simulink model "DFPD_DA_MdlIdent"  (R2017a)
settings: Solver=VariableStepAuto  StartTime=0.0  StopTime=190  FixedStep=0.001  RelTol=1e-3  EnableMultiTasking=on
PostLoadFcn:
  | , if any(exist('dsrtsu_mdlpostloadfcn', 'file') == [2, 3, 6]), try dsrtsu_mdlpostloadfcn('Execute', bdroot); catch fprintf('Error in PostLoadFcn (dsrtsu_mdlpostloadfcn) for model "%s":\n %s\n', bdroot, lasterr); end, end,
undefined symbols (not defined in the file or in its folder): DFPD_DoubleActing, mdlPara, PASL_Models
libraries: PASL_Mechanics x3, PASL_Pneumatics x3, PASL_Components x2, PASL_Tools x2
settings Model: DSRTSU_INTERNAL_RTI_VER=500  DSRTSU_INTERNAL_RTI_TYPE=rti1401  DSRTSU_INTERNAL_RTIFPGA=90  Creator=fbwk  LastModifiedBy=fbwk
settings DataIOCC: LimitDataPoints=on  SaveFormat=Array
settings OptimizationCC: BlockReduction=off  OptimizeBlockIOStorage=off  BufferReuse=off  GlobalBufferReuse=off  ExpressionFolding=off  LocalBlockOutputs=off  LifeSpan=inf
settings DebuggingCC: SolverPrmCheckMsg=warning  SFUnexpectedBacktrackingDiag=warning  SFNoUnconditionalDefaultTransitionDiag=warning  SFExecutionAtInitializationDiag=none
settings HardwareCC: ProdBitPerPointer=32  ProdBitPerSizeT=32  ProdBitPerPtrDiffT=32  ProdLargestAtomicInteger=Integer  ProdEndianess=BigEndian  ProdWordSize=32  ProdHWDeviceType=Custom Processor->Custom  TargetIntDivRoundTo=Zero  TargetEndianess=BigEndian  TargetHWDeviceType=Custom Processor->Custom
settings ModelReferenceCC: PropagateSignalLabelsOutOfModel=off
settings SFSimCC: MATLABDynamicMemAlloc=off
settings RTWCC: SystemTargetFile=rti1005.tlc  MakeCommand=make_rti  TemplateMakefile=rti1005.tmf  Description=dSPACE DS1005 Hardware Platform
settings STFCustomTargetCC: ParMdlRefBuildCompliant=on  MatFileLogging=on  GRTInterface=off  SystemTargetFile=rti1005.tlc
settings GRTTargetCC: TargetLangStandard=C89/C90 (ANSI)  CompOptLevelCompliant=off  ConcurrentExecutionCompliant=off  CombineOutputUpdateFcns=off  CPPClassGenCompliant=off  UseToolchainInfoCompliant=off  ExtModeMexFile=noextcomm
settings ConfigComp: CovMetricSettings=dw  CovHtmlReporting=on  CovSaveCumulativeToWorkspaceVar=on  CovSaveSingleToWorkspaceVar=on  CovExternalEMLEnable=off  CovSFcnEnable=off

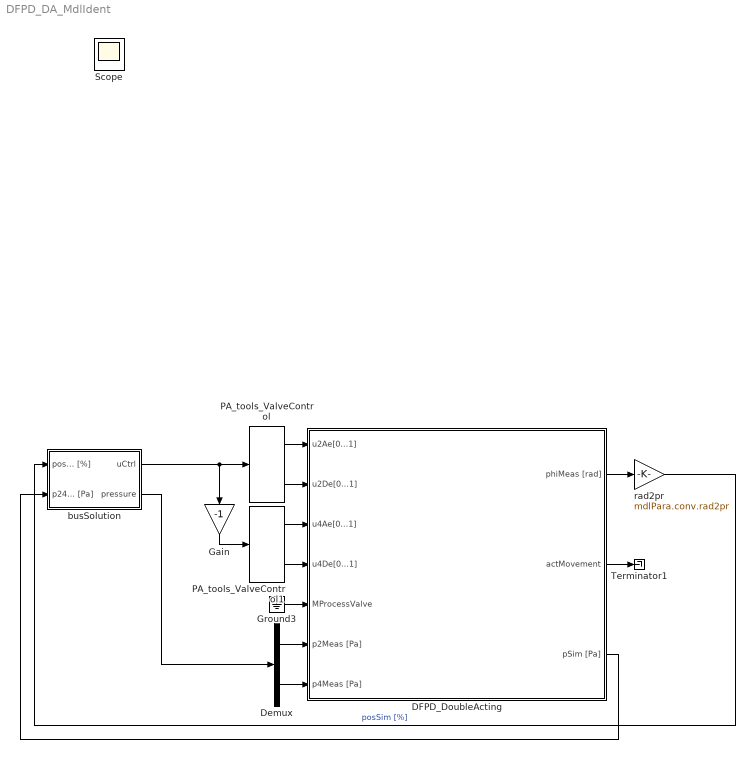
== system DFPD_DA_MdlIdent ==
  DFPD_DoubleActing : Subsystem  AncestorBlock=PASL_Models/DFPD_DoubleActing  TreatAsAtomicUnit=on  mask(Doppeltwirkender DFPD){mdlPara=mdlPara}
      mask prompts: mdlPara "Name of the parameters struct:"
      mask help:
      | Dieses Subsystem beinhaltet das Modell eines
      | doppeltwirkenden DFPDs.
      | Zur Initialisierung des Systems kann entweder
      | a) ein vorhandener Parametersatz geladen werden
      | oder
      | b) ein default Datensatz generiert werden.
      | Dabei werden die Daten des DFPD abgefragt
      | und alle aus der Konstruktion bekannten
      | Parameter entsprechend berechnet.
      |
      | !!Bisher ist das Reibungsmodell von Zahnstange
      | und Ritzel mit den Defaultwerten parametriert!!!
      |
      | 2016-09-20, lusc
      mask DialogControl Container4 Prompt: Parameter
      mask DialogControl Control5 Prompt: Parametersatz laden
      mask DialogControl Control5 Callback:
      | %% Modellparameter laden %%%%%%%%%%%%%%%%%%%%%%%%%%%%%%%%%%%%%%%%%%%%%%%%%%
      | 
      | % get mask parameters
      | maskval = get_param(gcb,'MaskValues');
      | structName = maskval{1};
      | 
      | % load parameters
      | assignin('base',structName,...
      | 	mdlPara = aux_loadMdlPara('DFPD')...
      | 	);
      | 
      | % clear section
      | clear maskval structName
      mask DialogControl Control6 Prompt: Parametersatz generieren
      mask DialogControl Control6 Callback:
      | %% Modellparameter laden %%%%%%%%%%%%%%%%%%%%%%%%%%%%%%%%%%%%%%%%%%%%%%%%%%
      | 
      | % get mask parameters
      | maskval = get_param(gcb,'MaskValues');
      | structName = maskval{1};
      | 
      | % load parameters
      | assignin('base',structName,aux_initMdlParaDFPD_DA());
      | 
      | % clear section
      | clear maskval structName
      mask Display:
      | image('DFPD_DoubleActing.jpg')
      | 
      | color('black')
      | port_label('input',1,'u2Ae [0...1]')
      | port_label('input',2,'u2De [0...1]')
      | port_label('input',3,'u4Ae [0...1]')
      | port_label('input',4,'u4De [0...1]')
      | port_label('input',5,'MProcessValve')
      | port_label('input',6,'p2 [Pa] (optional)')
      | port_label('input',7,'p4 [Pa] (optional)')
      | 
      | port_label('output',1,'phiMeas [rad]')
      | port_label('output',2,'actMovement')
  Demux : Demux  Outputs=2
  Gain : Gain  Gain=-1
  Ground3 : Ground
  PA_tools_ValveControl : PASL_Tools/PA_tools_ValveControl
      settings: SourceProductName=PASL
  PA_tools_ValveControl1 : PASL_Tools/PA_tools_ValveControl
      settings: SourceProductName=PASL
  Terminator1 : Terminator
  busSolution : Subsystem  VariantControl=busVariant
  rad2pr : Gain  Gain=mdlPara.conv.rad2pr
  Scope : Scope
  wires:
  busSolution/1(uCtrl) -> PA_tools_ValveControl/1, Gain/1
  Ground3/1 -> DFPD_DoubleActing/5("MProcessValve ")
  Demux/1 -> DFPD_DoubleActing/6(p2Meas [Pa])
  Demux/2 -> DFPD_DoubleActing/7(p4Meas [Pa])
  DFPD_DoubleActing/2(actMovement) -> Terminator1/1
  PA_tools_ValveControl/1 -> DFPD_DoubleActing/1(u2Ae[0...1])
  PA_tools_ValveControl/2 -> DFPD_DoubleActing/2(u2De[0...1])
  PA_tools_ValveControl1/1 -> DFPD_DoubleActing/3(u4Ae[0...1])
  PA_tools_ValveControl1/2 -> DFPD_DoubleActing/4(u4De[0...1])
  Gain/1 -> PA_tools_ValveControl1/1
  DFPD_DoubleActing/1(phiMeas [rad]) -> rad2pr/1
  busSolution/2(pressure) -> Demux/1
  DFPD_DoubleActing/3(pSim [Pa]) -> busSolution/2(p24Sim [Pa])
  rad2pr/1 -> busSolution/1(posSim [%])  "posSim [%]"

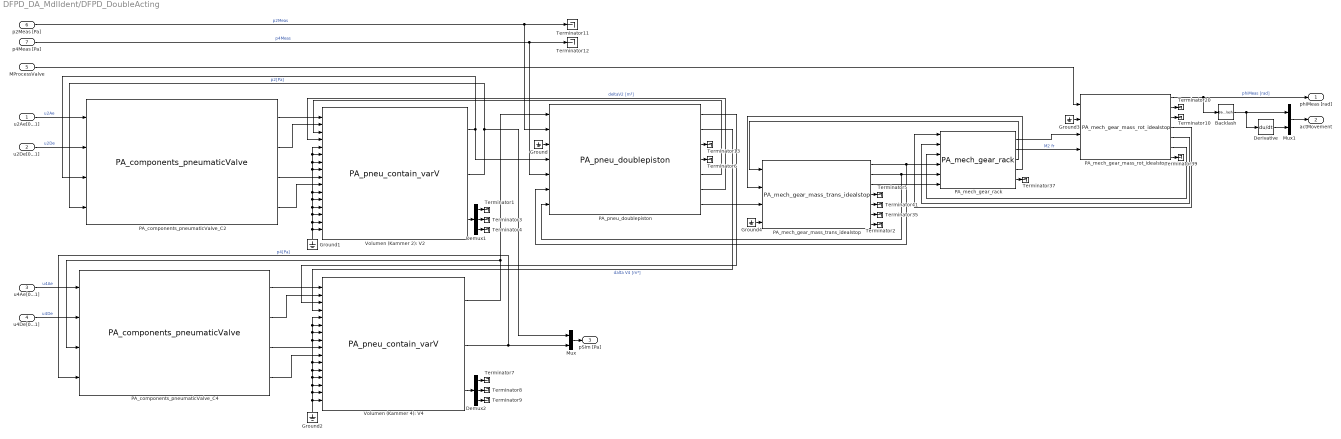
== system DFPD_DA_MdlIdent/DFPD_DoubleActing ==
  u2Ae[0...1] : Inport
  u2De[0...1] : Inport  Port=2
  u4Ae[0...1] : Inport  Port=3
  u4De[0...1] : Inport  Port=4
  "MProcessValve " : Inport  Port=5
  p2Meas [Pa] : Inport  Port=6
  p4Meas [Pa] : Inport  Port=7
  Backlash : Backlash  BacklashWidth=mdlPara.backlash
  Demux1 : Demux  Outputs=3
  Demux2 : Demux  Outputs=3
  Derivative : Derivative
  Ground{,1..4} (5 alike) : Ground
  Mux : Mux  Inputs=2
  Mux1 : Mux  Inputs=2
  PA_components_pneumaticValve_C2 : PASL_Components/PA_components_pneumaticValve  b=mdlPara.b  C=mdlPara.C2  pv=mdlPara.pv  pu=mdlPara.pu  Tu=mdlPara.Tu  R=mdlPara.R  n=mdlPara.n  smoothFact=mdlPara.smoothFac
      settings: SourceProductName=PASL
  PA_components_pneumaticValve_C4 : PASL_Components/PA_components_pneumaticValve  b=mdlPara.b  C=mdlPara.C4  pv=mdlPara.pv  pu=mdlPara.pu  Tu=mdlPara.Tu  R=mdlPara.R  n=mdlPara.n  smoothFact=mdlPara.smoothFac
      settings: SourceProductName=PASL
  PA_mech_gear_mass_rot_idealstop : PASL_Mechanics/Gear Elements/PA_mech_gear_mass_rot_idealstop  Tag=RB_mech_gear_mass_rot_idealstop  phiinit=mdlPara.phi0  phidotinit=mdlPara.phiDot0  J=mdlPara.inertia  drot1=mdlPara.pinionViscFri  drot2=0.0  drot3=0.0  phidotstri=mdlPara.pinionStribeckVel  Mstick=mdlPara.pinionMstick  Mslip=mdlPara.pinionMcoulomb  phimin=mdlPara.phiMin  phimax=mdlPara.phiMax
      settings: SourceProductName=PASL
  PA_mech_gear_mass_trans_idealstop : PASL_Mechanics/Gear Elements/PA_mech_gear_mass_trans_idealstop  Tag=RB_mech_gear_mass_rot_idealstop  xinit=mdlPara.x0  xdotinit=mdlPara.v0  m=mdlPara.mass  dtrans1=mdlPara.viscFriCoeff1  dtrans2=0.0  dtrans3=0.0  xdotstri=mdlPara.stribeckVel  Fstick=mdlPara.Fstick  Fslip=mdlPara.Fcoulomb  xmin=mdlPara.xMin  xmax=mdlPara.xMax
      settings: SourceProductName=PASL
  PA_mech_gear_rack : PASL_Mechanics/Gear Elements/PA_mech_gear_rack  Tag=RB_mech_gear_rack_partrans  r2=mdlPara.pitchRadius  lot=mdlPara.lot  dx0=mdlPara.initRelShift  cgeartrans=mdlPara.gearStiffness  dgeartrans=mdlPara.gearDamp  Fdmax=mdlPara.maxDampForce  eta=mdlPara.eta  etamode=mode 1: robust
      settings: SourceProductName=PASL
  PA_pneu_doublepiston : PASL_Pneumatics/Pistons/PA_pneu_doublepiston  d_out2=mdlPara.d4Out  d_in2=mdlPara.d4In  d_out4=mdlPara.d2Out  d_in4=mdlPara.d2In  x_02=mdlPara.x04  x_04=mdlPara.x02  p0=mdlPara.pu
      settings: SourceProductName=PASL
  Terminator{1..13,20,35,37,39,41} (18 alike) : Terminator
  Volumen (Kammer 2): V2 : PASL_Pneumatics/Volumes/PA_pneu_contain_varV  p0=mdlPara.p02  T0=mdlPara.Tu  V0=mdlPara.V02  K=mdlPara.heatExCoeff  A=mdlPara.heatExArea  Tw=mdlPara.Tu  R=mdlPara.R  kappa=mdlPara.n  temp_effects=without temperature effects
      settings: SourceProductName=PASL
  Volumen (Kammer 4): V4 : PASL_Pneumatics/Volumes/PA_pneu_contain_varV  p0=mdlPara.p04  T0=mdlPara.Tu  V0=mdlPara.V04  K=mdlPara.heatExCoeff  A=mdlPara.heatExArea  Tw=mdlPara.Tu  R=mdlPara.R  kappa=mdlPara.n  temp_effects=without temperature effects
      settings: SourceProductName=PASL
  phiMeas [rad] : Outport
  actMovement : Outport  Port=2
  pSim [Pa] : Outport  Port=3
  wires:
  Demux2/3 -> Terminator9/1
  Demux2/2 -> Terminator8/1
  Demux2/1 -> Terminator7/1
  Mux1/1 -> actMovement/1
  Derivative/1 -> Mux1/2
  Backlash/1 -> Derivative/1, Mux1/1
  PA_mech_gear_mass_rot_idealstop/2 -> Terminator20/1
  PA_mech_gear_mass_rot_idealstop/3 -> Terminator10/1
  PA_mech_gear_mass_rot_idealstop/1 -> phiMeas [rad]/1, Backlash/1  "phiMeas [rad]"
  PA_pneu_doublepiston/7 -> PA_mech_gear_mass_trans_idealstop/3
  "MProcessValve "/1 -> PA_mech_gear_mass_rot_idealstop/1
  Volumen (Kammer 4): V4/1 -> PA_pneu_doublepiston/1, PA_components_pneumaticValve_C4/3
  Ground/1 -> PA_pneu_doublepiston/3
  PA_pneu_doublepiston/4 -> Terminator6/1
  PA_pneu_doublepiston/3 -> Terminator13/1
  PA_pneu_doublepiston/2 -> Volumen (Kammer 4): V4/4  "dalta V4 [m³]"
  PA_pneu_doublepiston/1 -> Volumen (Kammer 4): V4/3
  PA_pneu_doublepiston/5 -> Volumen (Kammer 2): V2/3
  Demux1/3 -> Terminator4/1
  Demux1/2 -> Terminator3/1
  Volumen (Kammer 4): V4/3 -> Demux2/1
  Demux1/1 -> Terminator1/1
  Volumen (Kammer 2): V2/3 -> Demux1/1
  Ground2/1 -> Volumen (Kammer 4): V4/16, Volumen (Kammer 4): V4/7, Volumen (Kammer 4): V4/5, Volumen (Kammer 4): V4/6, Volumen (Kammer 4): V4/8, Volumen (Kammer 4): V4/11, Volumen (Kammer 4): V4/12, Volumen (Kammer 4): V4/13, Volumen (Kammer 4): V4/14, Volumen (Kammer 4): V4/15
  Volumen (Kammer 4): V4/2 -> PA_components_pneumaticValve_C4/4, Mux/2  "p4[Pa]"
  PA_pneu_doublepiston/6 -> Volumen (Kammer 2): V2/4  "deltaV2 [m³]"
  Ground1/1 -> Volumen (Kammer 2): V2/5, Volumen (Kammer 2): V2/6, Volumen (Kammer 2): V2/7, Volumen (Kammer 2): V2/8, Volumen (Kammer 2): V2/11, Volumen (Kammer 2): V2/12, Volumen (Kammer 2): V2/13, Volumen (Kammer 2): V2/14, Volumen (Kammer 2): V2/15, Volumen (Kammer 2): V2/16
  Volumen (Kammer 2): V2/2 -> Mux/1, PA_components_pneumaticValve_C2/4  "p2[Pa]"
  Volumen (Kammer 2): V2/1 -> PA_pneu_doublepiston/4, PA_components_pneumaticValve_C2/3
  PA_mech_gear_rack/2 -> PA_mech_gear_mass_rot_idealstop/4  "M2 fr"
  Ground3/1 -> PA_mech_gear_mass_rot_idealstop/2
  PA_mech_gear_mass_rot_idealstop/7 -> Terminator39/1
  Ground4/1 -> PA_mech_gear_mass_trans_idealstop/4
  PA_mech_gear_mass_trans_idealstop/4 -> Terminator5/1
  PA_mech_gear_mass_trans_idealstop/5 -> Terminator41/1
  PA_mech_gear_mass_trans_idealstop/6 -> Terminator35/1
  PA_mech_gear_rack/4 -> PA_mech_gear_mass_trans_idealstop/2
  PA_mech_gear_rack/3 -> PA_mech_gear_mass_trans_idealstop/1
  PA_mech_gear_mass_trans_idealstop/2 -> PA_pneu_doublepiston/7, PA_mech_gear_rack/5
  PA_mech_gear_mass_trans_idealstop/1 -> PA_pneu_doublepiston/6, PA_mech_gear_rack/4
  PA_mech_gear_rack/1 -> PA_mech_gear_mass_rot_idealstop/3
  PA_mech_gear_mass_trans_idealstop/7 -> Terminator2/1
  PA_mech_gear_rack/5 -> Terminator37/1
  PA_mech_gear_mass_rot_idealstop/5 -> PA_mech_gear_rack/2
  PA_mech_gear_mass_rot_idealstop/4 -> PA_mech_gear_rack/1
  PA_mech_gear_mass_rot_idealstop/6 -> PA_mech_gear_rack/3
  PA_mech_gear_mass_trans_idealstop/3 -> PA_mech_gear_rack/6
  PA_components_pneumaticValve_C4/1 -> Volumen (Kammer 4): V4/1
  PA_components_pneumaticValve_C4/2 -> Volumen (Kammer 4): V4/2
  PA_components_pneumaticValve_C4/3 -> Volumen (Kammer 4): V4/9
  PA_components_pneumaticValve_C4/4 -> Volumen (Kammer 4): V4/10
  PA_components_pneumaticValve_C2/1 -> Volumen (Kammer 2): V2/1
  PA_components_pneumaticValve_C2/2 -> Volumen (Kammer 2): V2/2
  PA_components_pneumaticValve_C2/3 -> Volumen (Kammer 2): V2/9
  PA_components_pneumaticValve_C2/4 -> Volumen (Kammer 2): V2/10
  p4Meas [Pa]/1 -> PA_pneu_doublepiston/5, Terminator12/1  "p4Meas"
  p2Meas [Pa]/1 -> PA_pneu_doublepiston/2, Terminator11/1  "p2Meas"
  u4De[0...1]/1 -> PA_components_pneumaticValve_C4/2  "u4De"
  u4Ae[0...1]/1 -> PA_components_pneumaticValve_C4/1  "u4Ae"
  u2De[0...1]/1 -> PA_components_pneumaticValve_C2/2  "u2De"
  u2Ae[0...1]/1 -> PA_components_pneumaticValve_C2/1  "u2Ae"
  Mux/1 -> pSim [Pa]/1

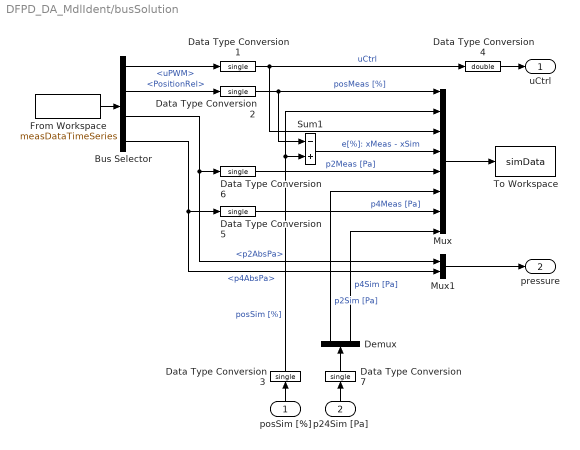
== system DFPD_DA_MdlIdent/busSolution ==
  posSim [%] : Inport
  p24Sim [Pa] : Inport  Port=2
  Bus Selector : BusSelector  OutputSignals=uPWM,PositionRel,p2AbsPa,p4AbsPa
  Data Type Conversion{1..3,5..7} (6 alike) : DataTypeConversion  OutDataTypeStr=single
  Data Type Conversion4 : DataTypeConversion  OutDataTypeStr=double
  Demux : Demux  Outputs=2
  From Workspace : FromWorkspace  VariableName=measDataTimeSeries  OutDataTypeStr=Bus: busMeasData  SampleTime=0
  Mux : Mux  Inputs=8
  Mux1 : Mux  Inputs=2
  Sum1 : Sum  Inputs=-+
  To Workspace : ToWorkspace  VariableName=simData  SaveFormat=Structure With Time  SampleTime=-1
  uCtrl : Outport
  pressure : Outport  Port=2
  wires:
  Data Type Conversion4/1 -> uCtrl/1
  Data Type Conversion3/1 -> Mux/2, Sum1/2  "posSim [%]"
  Data Type Conversion2/1 -> Sum1/1, Mux/1  "posMeas [%]"
  Data Type Conversion1/1 -> Data Type Conversion4/1, Mux/3  "uCtrl"
  Mux/1 -> To Workspace/1
  Sum1/1 -> Mux/4  "e[%]: xMeas - xSim"
  posSim [%]/1 -> Data Type Conversion3/1
  Bus Selector/2 -> Data Type Conversion2/1  "<PositionRel>"
  From Workspace/1 -> Bus Selector/1
  Bus Selector/1 -> Data Type Conversion1/1  "<uPWM>"
  Bus Selector/3 -> Mux1/1, Data Type Conversion6/1  "<p2AbsPa>"
  Bus Selector/4 -> Data Type Conversion5/1, Mux1/2  "<p4AbsPa>"
  Mux1/1 -> pressure/1
  p24Sim [Pa]/1 -> Data Type Conversion7/1
  Demux/1 -> Mux/6  "p2Sim [Pa]"
  Data Type Conversion6/1 -> Mux/5  "p2Meas [Pa]"
  Demux/2 -> Mux/8  "p4Sim [Pa]"
  Data Type Conversion7/1 -> Demux/1
  Data Type Conversion5/1 -> Mux/7  "p4Meas [Pa]"
